simulink model "Single_Phase_Inverter_B3"  (R2015a)
settings: Solver=ode45  StartTime=0.0  StopTime=0.3  RelTol=1e-3
libraries: powerlib x11, simulink x2, powerlib_meascontrol x1
settings Model: CovModelRefEnable=off  Creator=Rangga  LastModifiedBy=Rangga Putra
settings DataIOCC: LimitDataPoints=off  SaveFormat=StructureWithTime
settings HardwareCC: ProdBitPerPointer=64  ProdLargestAtomicFloat=Float  ProdIntDivRoundTo=Zero  ProdEndianess=LittleEndian  ProdHWDeviceType=Specified
settings ModelReferenceCC: PropagateSignalLabelsOutOfModel=on

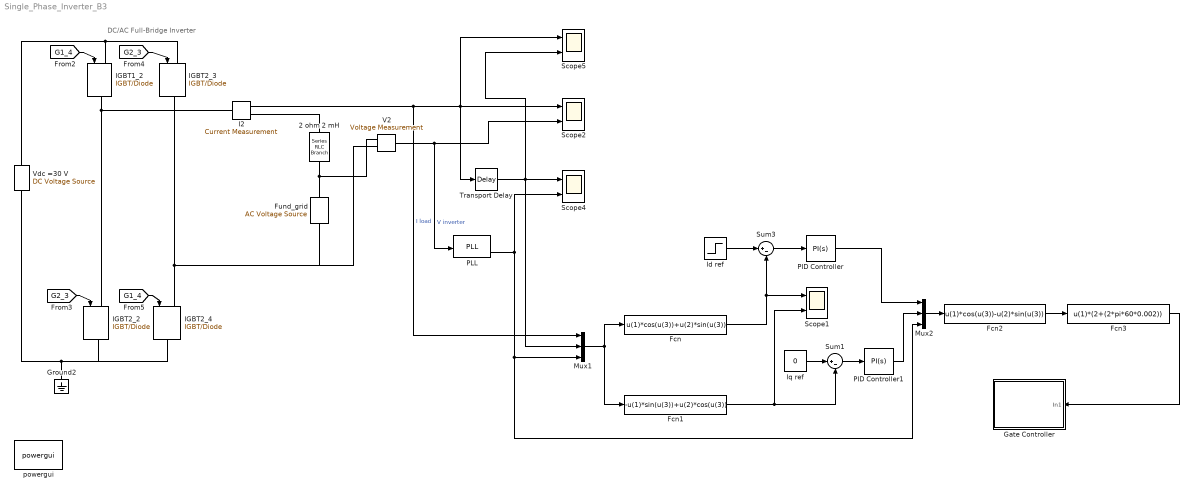
== system Single_Phase_Inverter_B3 ==
  note: DC/AC Full-Bridge Inverter
  "2 ohm 2 mH " : powerlib/Elements/Series RLC Branch  LConnTagsString=__new0  RConnTagsString=__new0  BranchType=RL  Resistance=2  Inductance=2e-3  SetiL0=off  InitialCurrent=0  Capacitance=[]  Setx0=off  InitialVoltage=0  Measurements=None
  Fcn : Fcn  Expr=u(1)*cos(u(3))+u(2)*sin(u(3))
  Fcn1 : Fcn  Expr=-u(1)*sin(u(3))+u(2)*cos(u(3))
  Fcn2 : Fcn  Expr=u(1)*cos(u(3))-u(2)*sin(u(3))
  Fcn3 : Fcn  Expr=u(1)*(2+(2*pi*60*0.002))
  Fund_grid : powerlib/Electrical Sources/AC Voltage Source  Amplitude=24  Phase=0  Frequency=60  SampleTime=0  Measurements=None
  Gate Controller : Subsystem
  Ground2 : powerlib/Elements/Ground  LConnTagsString=a
  I2 : powerlib/Measurements/Current Measurement  Tag=PoWeRsYsTeMmEaSuReMeNt  PhasorSimulation=off  OutputType=Magnitude  PSBequivalent=0
  IGBT1_2 : powerlib/Power Electronics/IGBT//Diode  Ron=1e-3  Rs=1e5  Cs=inf  Measurements=off
  IGBT2_2 : powerlib/Power Electronics/IGBT//Diode  Ron=1e-3  Rs=1e5  Cs=inf  Measurements=off
  IGBT2_3 : powerlib/Power Electronics/IGBT//Diode  Ron=1e-3  Rs=1e5  Cs=inf  Measurements=off
  IGBT2_4 : powerlib/Power Electronics/IGBT//Diode  Ron=1e-3  Rs=1e5  Cs=inf  Measurements=off
  Id ref : Step  Time=0.4  Before=50  After=100  SampleTime=5.144e-6
  Iq ref : Constant  Value=0
  Mux1 : Mux  Inputs=3
  Mux2 : Mux  Inputs=3
  PID Controller : simulink/Continuous/PID Controller  Controller=PI  TimeDomain=Continuous-time  SampleTime=-1  IntegratorMethod=Forward Euler  FilterMethod=Forward Euler  Form=Parallel  UseFilter=on  ControllerParametersSource=internal  P=1  I=1  D=0  N=100  InitialConditionSource=internal  InitialConditionForIntegrator=0  InitialConditionForFilter=0  ExternalReset=none  LimitOutput=off  UpperSaturationLimit=inf  LowerSaturationLimit=-inf  LinearizeAsGain=on  AntiWindupMode=none  Kb=1  TrackingMode=off  Kt=1  PParamMin=[]  PParamMax=[]  IParamMin=[]  IParamMax=[]  DParamMin=[]  DParamMax=[]  NParamMin=[]  NParamMax=[]  KbParamMin=[]  KbParamMax=[]  KtParamMin=[]  KtParamMax=[]  POutMin=[]  POutMax=[]  IOutMin=[]  IOutMax=[]  DOutMin=[]  DOutMax=[]  NOutMin=[]  NOutMax=[]  KbOutMin=[]  KbOutMax=[]  KtOutMin=[]  KtOutMax=[]  IntegratorOutMin=[]  IntegratorOutMax=[]  FilterOutMin=[]  FilterOutMax=[]  SumOutMin=[]  SumOutMax=[]  SumI1OutMin=[]  SumI1OutMax=[]  SumI2OutMin=[]  SumI2OutMax=[]  SumI3OutMin=[]  SumI3OutMax=[]  SumDOutMin=[]  SumDOutMax=[]  SaturationOutMin=[]  SaturationOutMax=[]  IntegratorContinuousStateAttributes=''  IntegratorStateMustResolveToSignalObject=off  IntegratorRTWStateStorageClass=Auto  FilterContinuousStateAttributes=''  FilterStateMustResolveToSignalObject=off  FilterRTWStateStorageClass=Auto  DifferentiatorICPrevScaledInput=0  DifferentiatorOutMin=[]  DifferentiatorOutMax=[]
  PID Controller1 : simulink/Continuous/PID Controller  Controller=PI  TimeDomain=Continuous-time  SampleTime=-1  IntegratorMethod=Forward Euler  FilterMethod=Forward Euler  Form=Parallel  UseFilter=on  ControllerParametersSource=internal  P=1  I=1  D=0  N=100  InitialConditionSource=internal  InitialConditionForIntegrator=0  InitialConditionForFilter=0  ExternalReset=none  LimitOutput=off  UpperSaturationLimit=inf  LowerSaturationLimit=-inf  LinearizeAsGain=on  AntiWindupMode=none  Kb=1  TrackingMode=off  Kt=1  PParamMin=[]  PParamMax=[]  IParamMin=[]  IParamMax=[]  DParamMin=[]  DParamMax=[]  NParamMin=[]  NParamMax=[]  KbParamMin=[]  KbParamMax=[]  KtParamMin=[]  KtParamMax=[]  POutMin=[]  POutMax=[]  IOutMin=[]  IOutMax=[]  DOutMin=[]  DOutMax=[]  NOutMin=[]  NOutMax=[]  KbOutMin=[]  KbOutMax=[]  KtOutMin=[]  KtOutMax=[]  IntegratorOutMin=[]  IntegratorOutMax=[]  FilterOutMin=[]  FilterOutMax=[]  SumOutMin=[]  SumOutMax=[]  SumI1OutMin=[]  SumI1OutMax=[]  SumI2OutMin=[]  SumI2OutMax=[]  SumI3OutMin=[]  SumI3OutMax=[]  SumDOutMin=[]  SumDOutMax=[]  SaturationOutMin=[]  SaturationOutMax=[]  IntegratorContinuousStateAttributes=''  IntegratorStateMustResolveToSignalObject=off  IntegratorRTWStateStorageClass=Auto  FilterContinuousStateAttributes=''  FilterStateMustResolveToSignalObject=off  FilterRTWStateStorageClass=Auto  DifferentiatorICPrevScaledInput=0  DifferentiatorOutMin=[]  DifferentiatorOutMax=[]
  PLL : powerlib_meascontrol/PLL/PLL  Fmin=45  Par_Init=[0, 60]  ParK=[180, 3200, 1]  TcD=1e-4  MaxRateChangeFreq=12  FilterCutOffFreq=25  Ts=0  AGC=on
  Scope{1..2,4..5} (4 alike) : Scope  NumInputPorts=2
      Scope1 settings: TimeRange=0.1  YMin=-9.43501~-5  YMax=9.4306~5  SaveName=ScopeData2
      Scope2 settings: TimeRange=0.1  YMin=-110~-225  YMax=110~225
      Scope4 settings: TimeRange=0.1  YMin=-9.48693~-21.49837  YMax=9.50207~21.19871  SaveName=ScopeData3
      Scope5 settings: TimeRange=0.1  YMin=-9.43501~-5  YMax=9.4306~5  SaveName=ScopeData4
  Sum1 : Sum  Inputs=|+-
  Sum3 : Sum  Inputs=|+-
  Transport Delay : TransportDelay  DelayTime=1/240  BufferSize=2048
  V2 : powerlib/Measurements/Voltage Measurement  Tag=PoWeRsYsTeMmEaSuReMeNt  PhasorSimulation=off  OutputType=Magnitude  PSBequivalent=0
  Vdc =30 V : powerlib/Electrical Sources/DC Voltage Source  Description=source block  Amplitude=30  Measurements=None
      settings: AttributesFormatString=\n
  powergui : powerlib/powergui  Priority=1  SimulationMode=Continuous  SolverType=Tustin/Backward Euler (TBE)  SampleTime=1e-6  frequency=60  SPID=on  DisableSnubberDevices=off  DisableRonSwitches=off  DisableVfSwitches=off  SwTol=0  DisplayEquations=off  Interpol=off  methode=off  Ts=10  FunctionMessages=off  echomessages=off  HookPort=off  EnableUseOfTLC=off  x0status=blocks  frequencyindice=0  Pbase=100e6  ErrMax=1e-4  Iterations=50  UnitsV=kV  UnitsW=MW  buscounter=0  RestoreLinks=warning  ResistiveCurrentMeasurement=off  Frange=[0:2:500]  Ylog=off  Xlog=on  ShowGrid=off  save=off  variable=ZData  structure=Iout  ZoomFFT=on  StartTime=0.2  cycles=2  DisplayStyle=1  fundamental=60  FreqAxis=off  MaxFrequency=1000  frequencyindicesteady=1  RmsSteady=1  display=off
  wires:
  I2/1 -> Mux1/1, Transport Delay/1, Scope2/1, Scope5/1  "I load"
  [G1_4] -> IGBT1_2/1
  [G2_3] -> IGBT2_2/1
  [G2_3] -> IGBT2_3/1
  [G1_4] -> IGBT2_4/1
  V2/1 -> Scope2/2, PLL/1  "V inverter"
  PLL/2 -> Mux1/3, Mux2/3, Scope4/2
  Transport Delay/1 -> Mux1/2, Scope4/1, Scope5/2
  Mux1/1 -> Fcn1/1, Fcn/1
  Fcn/1 -> Scope1/1, Sum3/2
  Id ref/1 -> Sum3/1
  Fcn1/1 -> Scope1/2, Sum1/2
  Iq ref/1 -> Sum1/1
  Sum3/1 -> PID Controller/1
  Sum1/1 -> PID Controller1/1
  PID Controller/1 -> Mux2/1
  PID Controller1/1 -> Mux2/2
  Mux2/1 -> Fcn2/1
  Fcn2/1 -> Fcn3/1
  Fcn3/1 -> Gate Controller/1(In1)
  connections:
  I2/RConn1 -- "2 ohm 2 mH "/LConn1
  IGBT2_4/RConn1 -- IGBT2_2/RConn1 -- Vdc =30 V/LConn1 -- Ground2/LConn1
  Vdc =30 V/RConn1 -- IGBT1_2/LConn1 -- IGBT2_3/LConn1
  IGBT1_2/RConn1 -- I2/LConn1 -- IGBT2_2/LConn1
  IGBT2_3/RConn1 -- Fund_grid/LConn1 -- V2/LConn2 -- IGBT2_4/LConn1
  "2 ohm 2 mH "/RConn1 -- V2/LConn1 -- Fund_grid/RConn1

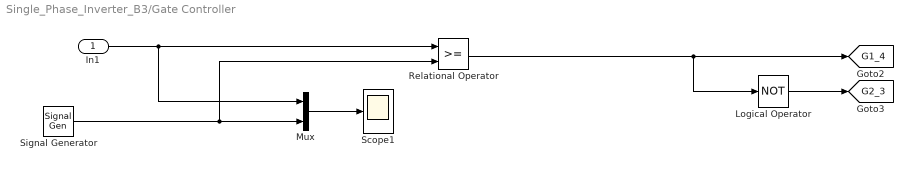
== system Single_Phase_Inverter_B3/Gate Controller ==
  In1 : Inport
  Logical Operator : Logic  Operator=NOT  AllPortsSameDT=off  OutDataTypeStr=boolean
  Mux : Mux  Inputs=2
  Relational Operator : RelationalOperator  OutDataTypeStr=boolean
  Scope1 : Scope
      settings: TimeRange=0.1  YMin=-1.04909  YMax=1.05376
  Signal Generator : SignalGenerator  Amplitude=300  Frequency=10000  Units=rad/sec
  tag scope: G1_4=global, G2_3=global
  wires:
  Signal Generator/1 -> Mux/2, Relational Operator/2
  Relational Operator/1 -> Logical Operator/1, [G1_4]
  Logical Operator/1 -> [G2_3]
  In1/1 -> Mux/1, Relational Operator/1
  Mux/1 -> Scope1/1
